simulink model "simulation_file"  (R2023b)
settings: Solver=FixedStepAuto  StartTime=0.0  StopTime=16  FixedStep=0.001  RelTol=1e-3
InitFcn:
  | importfrankaEmikaPanda
values from neighbouring files (symbols this model uses):
  d_influence = 0.06    [distance_with_linesegments_test.m]    (also in importfrankaEmikaPanda.m; matlab_obstacle_avoidance.m = 0.04)
  d_stop = 0.02    [distance_with_linesegments_test.m]    (also in importfrankaEmikaPanda.m; matlab_obstacle_avoidance.m = 0.01)
  Gripper_orientation = [-pi/4 0 0]    [importfrankaEmikaPanda.m]
  Gripper_position = [0 0 0.103399]    [importfrankaEmikaPanda.m]
  Homejointpositions = [0 ,0, 0, -pi/2, 0, pi/2, pi/4]    [importfrankaEmikaPanda.m]
  jointMaxValues = [2.8973, 1.7628, 2.8973, -0.0698, 2.8973, 3.7525, 2.8973]    [importfrankaEmikaPanda.m]
  jointMinValues = [-2.8973, -1.7628, -2.8973, -3.0718, -2.8973, 0.6500, -2.8973]    [importfrankaEmikaPanda.m]
  jointvelMaxValues = [2.1750 2.1750 2.1750 2.1750 2.6100 2.6100 2.6100]    [importfrankaEmikaPanda.m]
  jointvelMinValues = [-2.1750 -2.1750 -2.1750 -2.1750 -2.6100 -2.6100 -2.6100]    [importfrankaEmikaPanda.m]
  m = sqrt(det(JJt))    [computeManipulabilityJacobian.m]
  maxWaypoints = 20    [createWaypointData.m]    (also in importfrankaEmikaPanda.m)
  mdhparams = [ ... (first row only)    [importfrankaEmikaPanda.m]
  obstacle_sphere_1 = struct(     'type', OBSTACLE_SPHERE,      'center', [0, 0.20, 0.8],      'dimensions', [0.1, 0.1, 0.1],      'orientation', [1, 0, 0, 0],      'axis', 0  )    [importfrankaEmikaPanda.m]    (also in matlab_obstacle_avoidance.m = struct(     'type', OBSTACLE_SPHERE,      'center', [0.5545,)
  orientations = [0     0    0 ... (first row only)    [createWaypointData.m]    (also in importfrankaEmikaPanda.m = orientations'; matlab_obstacle_avoidance.m = orientations')
  ts = 0.01    [createWaypointData.m]    (also in importfrankaEmikaPanda.m = 0.001; matlab_obstacle_avoidance.m = 0.001)
  waypointAccels = zeros(size(waypointVels))    [createWaypointData.m]    (also in importfrankaEmikaPanda.m; matlab_obstacle_avoidance.m)
  waypoints = toolPositionHome' +              [0 0 0 ; 0 0 0 ; 0 0 0 ; 0 0 0 ; 0 0 0]'    [createWaypointData.m]    (also in importfrankaEmikaPanda.m = waypoints'; matlab_obstacle_avoidance.m = waypoints')
  waypointTimes = 0:4:16    [createWaypointData.m]    (also in importfrankaEmikaPanda.m; matlab_obstacle_avoidance.m)
  waypointVels = 0.1 *[ 0  0  0 ... (first row only)    [createWaypointData.m]    (also in importfrankaEmikaPanda.m; matlab_obstacle_avoidance.m)
  X = X + v0(1)    [plotCylinder.m]    (also in plotCylinder_foranimation.m)
  Y = Y + v0(2)    [plotCylinder.m]    (also in plotCylinder_foranimation.m)
  Z = Z + v0(3)    [plotCylinder.m]    (also in plotCylinder_foranimation.m)
undefined symbols (not defined in the file or in its folder): diff
libraries: sm_lib x98, nesl_utility x15, robotmaniplib x11, trajExampleUtils x9, robotcorelib x7
(part 4 of 4)

== matlab function simulation_file/Configuration_parameters ==
  data: robot output; dhparams_out output; mdhparams_out output; jointMinValues_out output; jointMaxValues_out output; jointvelMinValues_out output; jointvelMaxValues_out output; Homejointpositions_out output; waypoints_out output; orientations_out output; waypointTimes output; ts output; trajTimes output; waypointVels output; waypointAccels output; waypointAccelTimes output; obstacles_out output; d_stop output; d_influence output; radius_of_linesegments output
function [robot,dhparams_out,mdhparams_out,jointMinValues_out,jointMaxValues_out,jointvelMinValues_out,...
    jointvelMaxValues_out,Homejointpositions_out,waypoints_out,orientations_out,waypointTimes,ts,trajTimes, ...
    waypointVels,waypointAccels,waypointAccelTimes, obstacles_out,d_stop,d_influence,radius_of_linesegments]  = configuration_parameters()


persistent mdhparams dhparams Homejointpositions
persistent frankarobot_mdh waypoints orientations
persistent jointMinValues Starting_tcp_tform
persistent jointMaxValues toolPositionHome
persistent jointvelMinValues obstacles
persistent jointvelMaxValues



% First column defines  a
% Second column defines alpha (rad)
% Thrid column defines d 
% fourths column is theta (rad) 
%   a      alpha     d   theta
if isempty(mdhparams)
mdhparams = [
    0       0       0.333   0;
    0       -pi/2   0       0;
    0       pi/2    0.316   0;
    0.0825  pi/2    0       0;
   -0.0825 -pi/2    0.384   0;
    0       pi/2    0       0;
    0.088   pi/2    0.107   0
];
end
mdhparams_out = mdhparams;

if isempty(dhparams)
dhparams = [
    0,      -pi/2,    0.333,  0;
    0,       pi/2,    0,      0;
    0.0825,  pi/2,    0.316,  0;
   -0.0825, -pi/2,    0,      0;
    0,       pi/2,    0.384,  0;
    0.088,   pi/2,    0,      0;
    0.0003,   0,    0.107,  0];
end
dhparams_out = dhparams;

if isempty(jointMinValues) && isempty(jointMaxValues)
    jointMinValues = [-2.8973, -1.7628, -2.8973, -3.0718, -2.8973, 0.6500, -2.8973];
    jointMaxValues = [2.8973, 1.7628, 2.8973, -0.0698, 2.8973, 3.7525, 2.8973];
end 
jointMinValues_out = jointMinValues;
jointMaxValues_out = jointMaxValues;

if isempty(jointvelMinValues) && isempty(jointvelMaxValues)
    jointvelMinValues = [-2.1750 -2.1750 -2.1750 -2.1750 -2.6100 -2.6100 -2.6100];
    jointvelMaxValues = [2.1750 2.1750 2.1750 2.1750 2.6100 2.6100 2.6100];
end 

jointvelMinValues_out = jointvelMinValues;
jointvelMaxValues_out = jointvelMaxValues;

if isempty(Homejointpositions)
    Homejointpositions = [0 ,0, 0, -pi/2, 0, pi/2, pi/4];
    %Homejointpositions = [0 ,0, 0, -0.08, 0, 0.7, 0];
end 
Homejointpositions_out =  Homejointpositions;
number_of_joints = length(mdhparams);
Gripper_position = [0 0 0.103399];
Gripper_orientation = [-pi/4 0 0];
frankarobot  = loadrobot("frankaEmikaPanda");
%show(frankarobot)
body_Tcp_2 = rigidBody('Gripper_TCP');
joint_Tcp_2 = rigidBodyJoint('Gripper_TCP_frame', 'fixed');
tform_tcp_2 = trvec2tform([0 0 0.103399])*eul2tform([-pi/4 0 0]);
setFixedTransform(joint_Tcp_2,tform_tcp_2);
body_Tcp_2.Joint = joint_Tcp_2;
addBody(frankarobot,body_Tcp_2,'panda_link8');

%Set initial joint position

 Initalconfig = frankarobot.homeConfiguration;
% 
 for i = 1:7
      Initalconfig(i).JointPosition = Homejointpositions(i);
 end
% 
% % Set the modified home configuration back to the robot



% cd ~/MATLAB/<version>
 
%Set End effector name + set TcP at Gripper
%BUild robot from mDH Parameters  [a alpha d theta] MOdiefied DH
if isempty(frankarobot_mdh)

    %Create a rigid body tree. This tree is initialized with a base coordinate frame to attach bodies to.
    frankarobot_mdh = rigidBodyTree(MaxNumBodies= 50,DataFormat="row");
    body1 =rigidBody('robot_link1');
    jnt1 = rigidBodyJoint('robot_joint1','revolute');
    jnt1.HomePosition = Homejointpositions(1);
    jnt1.PositionLimits = [jointMinValues(1), jointMaxValues(1)];
    setFixedTransform(jnt1,mdhparams(1,:),'mdh');
    body1.Joint = jnt1;

    %Add the first body to the tree.
    % Specify that you are attaching it to the base of the tree.
    % The fixed transform defined previously is from the base (parent) to the first body.
    addBody(frankarobot_mdh,body1,'base')


    % Dynamically create and add the rest of the bodies
    for i = 2:number_of_joints
        bodyName = sprintf('robot_link%d', int32(i));
        jointName = sprintf('robot_joint%d', int32(i));
        body = rigidBody(bodyName);
        joint = rigidBodyJoint(jointName, 'revolute');
        joint.HomePosition = Homejointpositions(i);
        joint.PositionLimits = [jointMinValues(i), jointMaxValues(i)];
        setFixedTransform(joint, mdhparams(i,:), 'mdh');
        body.Joint = joint;
        addBody(frankarobot_mdh, body, sprintf('robot_link%d', int32(i-1)));
    end

    body_Tcp = rigidBody('Gripper_TCP');
    joint_Tcp = rigidBodyJoint('Gripper_TCP_frame', 'fixed');
    tform_tcp = trvec2tform(Gripper_position)*eul2tform(Gripper_orientation);
    setFixedTransform(joint_Tcp,tform_tcp);
    body_Tcp.Joint = joint_Tcp;
    addBody(frankarobot_mdh,body_Tcp,sprintf('robot_link%d', int32(number_of_joints)));

end

robot = frankarobot_mdh;

%getTransform(frankarobot,Initalconfig,'panda_link8','panda_link0');
%Initalconfig_mdh = frankarobot_mdh.homeConfiguration;

% for i = 1:
%     Initalconfig_mdh(i).JointPosition = Homejointpositions(i);
% end

if isempty(Starting_tcp_tform)
Starting_tcp_tform = getTransform(frankarobot_mdh,frankarobot_mdh.homeConfiguration,'Gripper_TCP','base');
toolPositionHome = Starting_tcp_tform(1:3,4);
end 

%showdetails(frankarobot_mdh); %showdetails function does not support code generation
%Jacobi_MATRIX = jacobian_cartesian(frankarobot_mdh,[0,0,0,-1.570796326794897,0,1.570796326794897,0.785398163397448],8);

% Maximum number of waypoints (for Simulink)
%maxWaypoints = 20;

% Positions (X Y Z)
% Define waypoints
if isempty(waypoints)
waypoints = [toolPositionHome'; 
             toolPositionHome' + [0, 0.1 , 0]; 
             toolPositionHome' + [0, 0.1, -0.1]; 
             toolPositionHome' + [0, -0.1, -0.1]; 
             toolPositionHome']';

end
waypoints_out = waypoints;
% waypoints = [toolPositionHome'; 
%              toolPositionHome' + [0, 0 , 0]; 
%              toolPositionHome' + [0, 0, 0]; 
%              toolPositionHome' + [0, -0, 0]; 
%              toolPositionHome'];
% + [0, 0, 0.2]
% Ensure waypoints are transposed correctly for vertical concatenation

         
% Euler Angles (Z Y X) relative to the home orientation       
% orientations = [0     0    pi;
%                 0  0    3*pi/4; 
%                 0   0  pi/2;
%                 0   0    3*pi/4;
%                 0   0    pi]';   

if isempty(orientations)    
orientations = [0     0    pi;
                0  0    pi; 
                0   0  pi;
                0   0    pi;
                0   0    pi]';         
end 
orientations_out = orientations;
% Array of waypoint times
waypointTimes = 0:4:16;

% Trajectory sample time
ts = 0.001; %1 ms
trajTimes = 0:ts:waypointTimes(end);

%% Additional parameters

% Boundary conditions (for polynomial trajectories)
% Velocity (cubic and quintic)
% waypointVels = 0.1 *[ 0  1  0;
%                      -1  0  0;
%                       0 -1  0;
%                       1  0  0;
%                       0  1  0]';

waypointVels = 0.1 *[ 0  0  0;
                     0  0  0;
                      0 0  0;
                      0  0  0;
                      0  0  0]';
% Acceleration (quintic only)
waypointAccels = zeros(size(waypointVels));

% Acceleration times (trapezoidal only)
waypointAccelTimes = diff(waypointTimes)/4;



%create obstacles structures 
% Fields not used by a particular obstacle type will be ignored in C++
%{
obstacle = struct(...
    'type', '', ...               % An integer or enum to represent the type
    'center', [0, 0, 0], ...
    'dimensions', [0, 0, 0], ... % for spehre all three entries radius.Use
    %for both radius-height of [radius height/2 height/2]cylinder and
    %dimensions of box[xlim ylim zlim]
    
    'orientation', [1, 0, 0, 0], ... % Default orientation (no rotation)
    'axis', [0, 0, 1] ...         % Default axis forobstacle.axis cylinders
);
%}
% Use an enum or integer to represent the obstacle type for efficiency
OBSTACLE_SPHERE = 1;
% OBSTACLE_CYLINDER = 2;
% OBSTACLE_BOX = 3;

if isempty(obstacles)
obstacle_sphere_1 = struct(...
    'type', OBSTACLE_SPHERE, ...               
    'center', [0, 0.15, 0.8], ...
    'dimensions', [0.05, 0.05, 0.05], ... 
    'orientation', [1, 0, 0, 0], ... 
    'axis', NaN ...        
);
obstacles = [obstacle_sphere_1];
end 
obstacles_out = obstacles;
% obstacle_sphere_2 = struct(...
%     'type', OBSTACLE_SPHERE, ...               
%     'center', [0, -0.7, 0.8], ...
%     'dimensions', [0.05, 0.05, 0.1], ... 
%     'orientation', NaN, ... 
%     'axis', NaN ...        
% );
%obstacles = [obstacle_sphere_1 obstacle_sphere_2];

%radius for each link
radius_of_linesegments = [0.06 0.06 0.06 0.06 0.06 0.06 0.06];
d_influence = 0.06;
d_stop = 0.03;


end

== matlab function simulation_file/Manual INVERSE KINEMATICS BlOCK/MATLAB Function ==
  data: T input; translation output
function translation = extractTranslation(T)
    % Extract the translation vector from the transformation matrix
    translation = T(1:3,4);
end

== matlab function simulation_file/Manual INVERSE KINEMATICS BlOCK/Jacobimatrix_to_ith_link/MATLAB Function ==
  data: T01 input; Jacobimatrix output; T02 input; T03 input; T04 input; T05 input; T06 input; T07 input; T0tcp input; to_ith_link input
function Jacobimatrix = fcn(T01,T02,T03,T04,T05,T06,T07,T0tcp,to_ith_link)

%Array of transformation matrices 
T = {T01,T02,T03,T04,T05,T06,T07,T0tcp};

numJoints = 7; % Number of joints
J = zeros(6, numJoints); % Initialize Jacobian matrix with zeros
    if to_ith_link == 8 
        T_end_effector = T0tcp;
    else
    % Compute the transformation to the end-effector or to_ith_link
    T_end_effector = T07;
    end
    
    end_effector_position = T_end_effector(1:3, 4);

    for i = 1:to_ith_link-1
        % Get the transformation matrix from the base frame to the ith joint
        T_i = T{i};

        % Extract the z-axis of the ith joint in base frame coordinates
        z_i = T_i(1:3, 1:3) * [0; 0; 1];

        % Position of the ith joint in base frame coordinates
        d_i = T_i(1:3, 4);

        % Linear velocity contribution: cross product of z-axis with the vector from joint i to the end-effector
        Jv_i = cross(z_i, (end_effector_position - d_i));

        % Angular velocity contribution: simply the z-axis for revolute joints
        Jw_i = z_i;

        % Fill in the ith column of the Jacobian matrix for joint i
        J(1:3, i) = Jv_i; % Upper part for linear velocity
        J(4:6, i) = Jw_i; % Lower part for angular velocity
    end

    % Columns of Jacobian corresponding to joints beyond to_ith_link are already initialized to zero
    Jacobimatrix = J;
end

== matlab function simulation_file/Manual INVERSE KINEMATICS BlOCK/quaternion_error/MATLAB Function1 ==
  data: qd input; qe output; qc input; T_i input
function qe = computequatError(qd, qc,T_i)
    %Ensure the quaternions are normalized
    %     qd = qd / norm(qd);
    % qc = qc / norm(qc);

    % Compute the conjugate of the current orientation quaternion
    
    
    
     eta_d = qd(1);
    eta = qc(1);
    q = qc(2:4);
    q_d = qd(2:4);

   qerror = -eta_d * q + eta * q_d - cross(q_d, q);
    %qerror = eta_d * q - eta * q_d + cross(q_d, q);
    qe = T_i(1:3, 1:3) * (qerror)';
    
    
    
    % 
    % qc_conj = [qc(1), -qc(2), -qc(3), -qc(4)];
    % 
    % % Compute the quaternion error
    % qerror = quatmultiply(qd, qc_conj);
    % 
    % axang = quat2axang(qerror);
    % 
    % qe_ax = (axang(4) * axang(1:3))';
    % qe = T_i(1:3, 1:3) * qe_ax;
end






   %   eta_d = qd(1);
   %  eta = qc(1);
   %  q = qc(2:4);
   %  q_d = qd(2:4);
   % 
   % %qe = -eta_d * q + eta * q_d - cross(q_d, q);
   %  qe = eta_d * q - eta * q_d + cross(q_d, q);

== matlab function simulation_file/Manual INVERSE KINEMATICS BlOCK/quaternion_error/MATLAB Function2 ==
  data: T input; quat output
function quat = tmatrix2quat(T)

% Make sure the rotation matrix is 3x3
R = T(1:3, 1:3);

% Preallocate the quaternion
quat = zeros(1, 4);

% Calculate the trace of the matrix
tr = trace(R);

% Check the value of the trace
if tr > 0
    S = sqrt(tr + 1.0) * 2; % S=4*qw
    quat(1) = 0.25 * S;
    quat(2) = (R(3,2) - R(2,3)) / S;
    quat(3) = (R(1,3) - R(3,1)) / S;
    quat(4) = (R(2,1) - R(1,2)) / S;
elseif (R(1,1) > R(2,2)) && (R(1,1) > R(3,3))
    S = sqrt(1.0 + R(1,1) - R(2,2) - R(3,3)) * 2; % S=4*qx
    quat(1) = (R(3,2) - R(2,3)) / S;
    quat(2) = 0.25 * S;
    quat(3) = (R(1,2) + R(2,1)) / S;
    quat(4) = (R(1,3) + R(3,1)) / S;
elseif R(2,2) > R(3,3)
    S = sqrt(1.0 + R(2,2) - R(1,1) - R(3,3)) * 2; % S=4*qy
    quat(1) = (R(1,3) - R(3,1)) / S;
    quat(2) = (R(1,2) + R(2,1)) / S;
    quat(3) = 0.25 * S;
    quat(4) = (R(2,3) + R(3,2)) / S;
else
    S = sqrt(1.0 + R(3,3) - R(1,1) - R(2,2)) * 2; % S=4*qz
    quat(1) = (R(2,1) - R(1,2)) / S;
    quat(2) = (R(1,3) + R(3,1)) / S;
    quat(3) = (R(2,3) + R(3,2)) / S;
    quat(4) = 0.25 * S;
end

% Normalize the quaternion
quat = quat / norm(quat);
end

== matlab function simulation_file/Manual INVERSE KINEMATICS BlOCK/MATLAB Function3 ==
  data: q_err input; omega output; delta_t input; T_i input
function omega = quatErrorToAngVel(q_err, delta_t,T_i)
    % Extract the scalar and vector parts from the quaternion error
    w = q_err(1);
    vec = q_err(2:4);

    % Ensure the scalar part of the quaternion is within the range [0, 1]
    w = max(min(w, 1), -1);

    % Calculate the rotation angle from the quaternion scalar part
    theta = 2 * acos(w);

    % Adjust theta to be in the range [0, pi]
    if theta > pi
        theta = 2 * pi - theta;
        vec = -vec; % Reverse the vector part if angle is greater than 180 degrees
    end

    % Calculate sin(theta/2)
    sin_half_theta = sin(theta / 2);

    % Prevent division by zero for small angles
    if abs(sin_half_theta) < eps
        omega = zeros(3, 1); % For small angles, omega is effectively zero
    else
        % For larger angles, calculate the angular velocity
        omega = theta / delta_t * (vec / sin_half_theta);
    end
end

== matlab function simulation_file/Trajectory Generation/Rotation Trajectory/Get Trajectory Index ==
  data: hasChanged output; t input; segIdx output; waypointTimes input size=[1 maxWaypoints]
function [hasChanged,segIdx] = getTrajIdx(t,waypointTimes)

% Initialize previous index
persistent prevIdx
if isempty(prevIdx)
    prevIdx = 0;
end

% Find the trajectory segment index
segIndices = find(t>=waypointTimes);

% Limit the index value to the number of times minus one
% (This addresses the final time case)
segIdx = min(segIndices(end),numel(waypointTimes)-1);

% Determine whether the index has changed from the previous time step
if prevIdx == segIdx
    hasChanged = false;
else
    hasChanged = true;
    prevIdx = segIdx;
end

end

== matlab function simulation_file/Trajectory Generation/Rotation Trajectory/Extract Trajectory Segment/MATLAB Function ==
  data: segIdx input; waypointTimes input size=[1 maxWaypoints]; q0 output size=[1 4]; orientations input size=[3 maxWaypoints]; qf output size=[1 4]; timeInterval output size=[1 2]
function [q0, qf, timeInterval] = createRotationTrajSegment(segIdx,waypointTimes,orientations)

% Extract the time interval, initial, and final quaternions for the segment
timeInterval = waypointTimes(segIdx:segIdx+1);
q0 = eul2quat(orientations(:,segIdx)');
qf = eul2quat(orientations(:,segIdx+1)');

end

== matlab function simulation_file/MATLAB Function4 ==
  data: jointvalues input; newjointvalues_withgripper output
function newjointvalues_withgripper = concatenatejoints(jointvalues)
newjointvalues_withgripper = zeros(9,1);
newjointvalues_withgripper(1:7) = jointvalues; 

end
